simulink model "Genset"  (R2019b)
settings: Solver=VariableStepAuto  StartTime=0.0  StopTime=tEnd  RelTol=1e-3
values from neighbouring files (symbols this model uses):
  etaGenGR = 0.93    [main.m]
  genMotorData = load(GENERATOR_MOTOR_DATA_NAME)    [main.m]
  GRgen = 1.4    [main.m]
  initialGasVolume = 5    [main.m]
  k_gal2kWh = 32.3    [main.m]
  k_hr2s = 3600    [main.m]
  k_m32gal = 264.172    [main.m]
  k_rpm2rps = 2*pi()/60    [main.m]
  k_W2kW = 1/1000    (= 0.001)    [main.m]
libraries: autolibsharedmappedengines x1
(part 3 of 3)

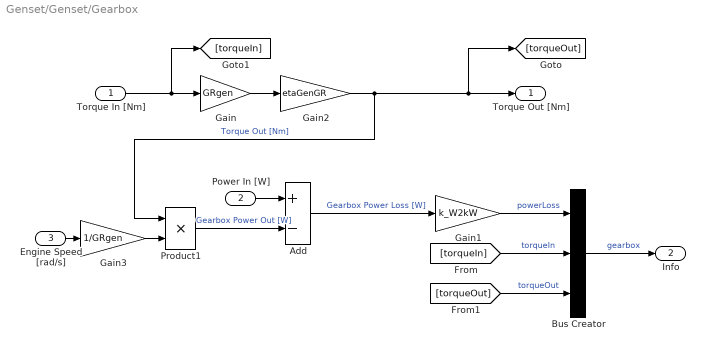
== system Genset/Genset/Gearbox ==
  Torque In [Nm] : Inport
  Power In [W] : Inport  Port=2
  Engine Speed [rad/s] : Inport  Port=3
  Add : Sum  Inputs=+-
  Bus Creator : BusCreator  Inputs=3
  Gain : Gain  Gain=GRgen
  Gain1 : Gain  Gain=k_W2kW
  Gain2 : Gain  Gain=etaGenGR
  Gain3 : Gain  Gain=1/GRgen
  Product1 : Product
  Torque Out [Nm] : Outport
  Info : Outport  Port=2
  wires:
  Gain2/1 -> [torqueOut], Torque Out [Nm]/1, Product1/1  "Torque Out [Nm]"
  Product1/1 -> Add/2  "Gearbox Power Out [W]"
  Engine Speed [rad/s]/1 -> Gain3/1
  Gain/1 -> Gain2/1
  Power In [W]/1 -> Add/1
  Add/1 -> Gain1/1  "Gearbox Power Loss [W]"
  Torque In [Nm]/1 -> [torqueIn], Gain/1
  Gain1/1 -> Bus Creator/1  "powerLoss"
  [torqueIn] -> Bus Creator/2  "torqueIn"
  [torqueOut] -> Bus Creator/3  "torqueOut"
  Bus Creator/1 -> Info/1  "gearbox"
  Gain3/1 -> Product1/2

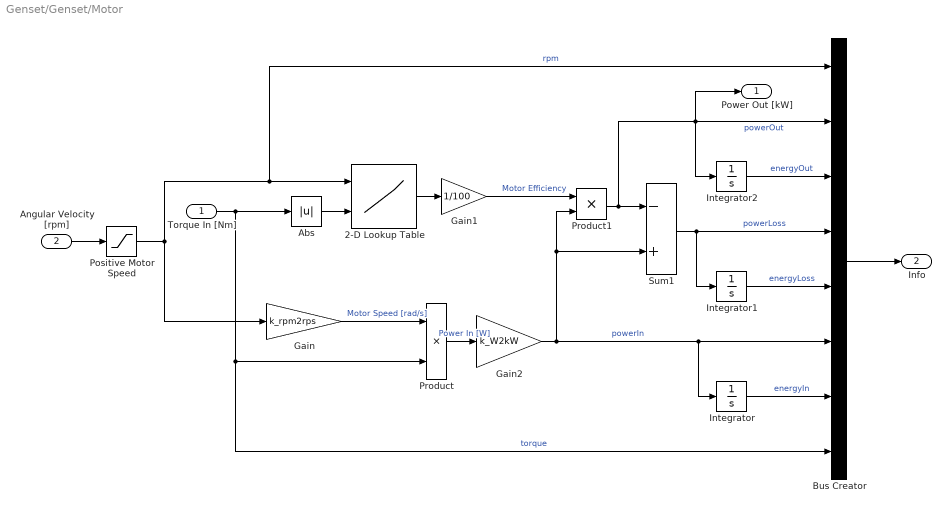
== system Genset/Genset/Motor ==
  Torque In [Nm] : Inport
  Angular Velocity [rpm] : Inport  Port=2
  2-D Lookup Table : Lookup_n-D  BreakpointsForDimension1=genMotorData.w_eff_bp  BreakpointsForDimension2=genMotorData.T_eff_bp  Table=genMotorData.efficiency_table  InternalRulePriority=Speed  RndMeth=Simplest  InputSameDT=on
  Abs : Abs
  Bus Creator : BusCreator  Inputs=8
  Gain : Gain  Gain=k_rpm2rps
  Gain1 : Gain  Gain=1/100
  Gain2 : Gain  Gain=k_W2kW
  Integrator : Integrator
  Integrator1 : Integrator
  Integrator2 : Integrator
  Positive Motor Speed : Saturate  UpperLimit=inf  LowerLimit=0
  Product : Product
  Product1 : Product
  Sum1 : Sum  Inputs=-+
  Power Out [kW] : Outport
  Info : Outport  Port=2
  wires:
  Angular Velocity [rpm]/1 -> Positive Motor Speed/1
  Gain/1 -> Product/1  "Motor Speed [rad/s]"
  Positive Motor Speed/1 -> Bus Creator/1, 2-D Lookup Table/1, Gain/1  "rpm"
  Gain1/1 -> Product1/1  "Motor Efficiency"
  Product1/1 -> Sum1/1, Power Out [kW]/1, Bus Creator/2, Integrator2/1  "powerOut"
  Integrator2/1 -> Bus Creator/3  "energyOut"
  Sum1/1 -> Bus Creator/4, Integrator1/1  "powerLoss"
  2-D Lookup Table/1 -> Gain1/1
  Abs/1 -> 2-D Lookup Table/2
  Integrator1/1 -> Bus Creator/5  "energyLoss"
  Integrator/1 -> Bus Creator/7  "energyIn"
  Torque In [Nm]/1 -> Abs/1, Bus Creator/8, Product/2  "torque"
  Gain2/1 -> Integrator/1, Bus Creator/6, Sum1/2, Product1/2  "powerIn"
  Bus Creator/1 -> Info/1
  Product/1 -> Gain2/1  "Power In [W]"
